simulink model "TASK7_2"  (R2019a)
settings: Solver=VariableStepAuto  StartTime=0.0  StopTime=30  RelTol=1e-3
values from neighbouring files (symbols this model uses):
  A = [0,mf*g*h/Jconst,0,-(mf*g)/Jconst;1,0,0,0;0,-g,0,0;0,0,1,0]    [Dharmesh_DCS_LAB_Script.m]
  B = [1/Jconst;0;0;0]    [Dharmesh_DCS_LAB_Script.m]
  C = eye(4)    [Dharmesh_DCS_LAB_Script.m]
  Ct = [0 0 0 1]    [Dharmesh_DCS_LAB_Script.m]
  D = [0;0;0;0]    [Dharmesh_DCS_LAB_Script.m]
  Ki = Kpi(1:4)-(P*Ct)    [Dharmesh_DCS_LAB_Script.m]
  Kt_o_new = Kt_o.'    [Dharmesh_DCS_LAB_Script.m]
  P = 1/(Ct*inv((B*K)-A)*B)    [Dharmesh_DCS_LAB_Script.m]
  Pi = -Kpi(5)    [Dharmesh_DCS_LAB_Script.m]
  Ts = 125e-6    (= 0.000125)    [Dharmesh_DCS_LAB_Script.m]
  x2 = [0;0;0;1]    [Dharmesh_DCS_LAB_Script.m]
undefined symbols (not defined in the file or in its folder): AD, BD
settings Model: Creator=Admin  LastModifiedBy=Admin

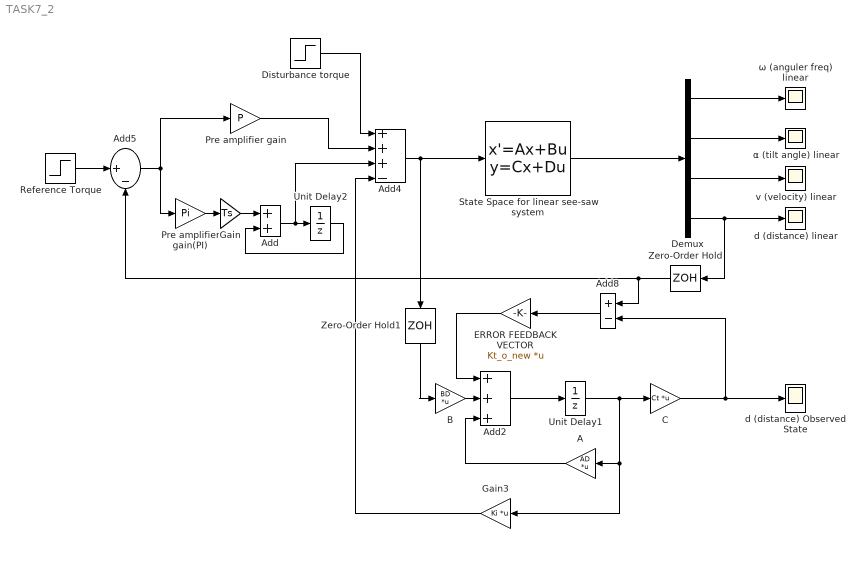
== system TASK7_2 ==
  A : Gain  Gain=AD  Multiplication=Matrix(K*u) (u vector)
  Add : Sum
  Add2 : Sum  Inputs=+++
  Add4 : Sum  Inputs=+++-
  Add5 : Sum  Inputs=|+-
  Add8 : Sum  Inputs=+-
  B : Gain  Gain=BD  Multiplication=Matrix(K*u) (u vector)
  C : Gain  Gain=Ct  Multiplication=Matrix(K*u) (u vector)
  Demux : Demux
  Disturbance torque : Step  Time=15  After=0.1  SampleTime=0
  ERROR FEEDBACK VECTOR : Gain  Gain=Kt_o_new  Multiplication=Matrix(K*u) (u vector)
  Gain : Gain  Gain=Ts
  Gain3 : Gain  Gain=Ki  Multiplication=Matrix(K*u) (u vector)
  Pre amplifier gain : Gain  Gain=P
  Pre amplifier gain(PI) : Gain  Gain=Pi
  Reference Torque : Step  Time=0  SampleTime=0
  State Space for linear see-saw system : StateSpace  A=A  B=B  C=C  D=D  InitialCondition=0
  Unit Delay1 : UnitDelay  InitialCondition=x2  SampleTime=Ts  HasFrameUpgradeWarning=on
  Unit Delay2 : UnitDelay  SampleTime=Ts  HasFrameUpgradeWarning=on
  Zero-Order Hold : ZeroOrderHold  SampleTime=Ts
  Zero-Order Hold1 : ZeroOrderHold  SampleTime=Ts
  d (distance) Observed State : Scope
  d (distance) linear : Scope
  v (velocity) linear : Scope
  α (tilt angle) linear : Scope
  ω (anguler freq) linear : Scope
  wires:
  C/1 -> d (distance) Observed State/1, Add8/2
  Reference Torque/1 -> Add5/1
  Demux/4 -> d (distance) linear/1, Zero-Order Hold/1
  Add4/1 -> Zero-Order Hold1/1, State Space for linear see-saw system/1
  Demux/3 -> v (velocity) linear/1
  Add5/1 -> Pre amplifier gain/1, Pre amplifier gain(PI)/1
  Demux/2 -> α (tilt angle) linear/1
  Demux/1 -> ω (anguler freq) linear/1
  State Space for linear see-saw system/1 -> Demux/1
  Disturbance torque/1 -> Add4/1
  Pre amplifier gain/1 -> Add4/2
  Add/1 -> Add4/3, Unit Delay2/1
  Add2/1 -> Unit Delay1/1
  Unit Delay1/1 -> A/1, Gain3/1, C/1
  Gain3/1 -> Add4/4
  Add8/1 -> ERROR FEEDBACK VECTOR/1
  A/1 -> Add2/3
  ERROR FEEDBACK VECTOR/1 -> Add2/1
  B/1 -> Add2/2
  Unit Delay2/1 -> Add/2
  Zero-Order Hold/1 -> Add8/1, Add5/2
  Zero-Order Hold1/1 -> B/1
  Pre amplifier gain(PI)/1 -> Gain/1
  Gain/1 -> Add/1
